simulink model "equation"  (R2025a)
settings: Solver=VariableStepAuto  StartTime=0.0  StopTime=10.0  RelTol=1e-3
settings Model: Creator=Johan  LastModifiedBy=Johan

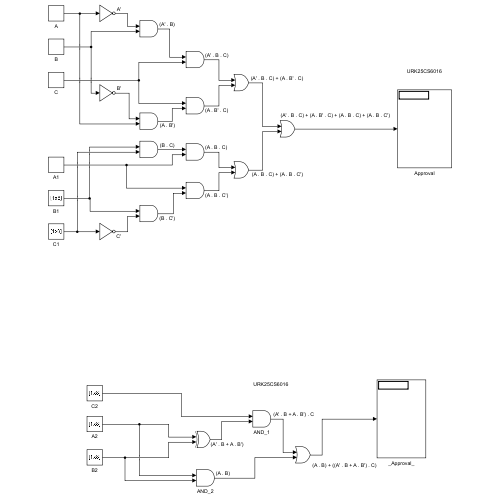
[thumbnail: Simulink's stored preview of the top-level diagram]
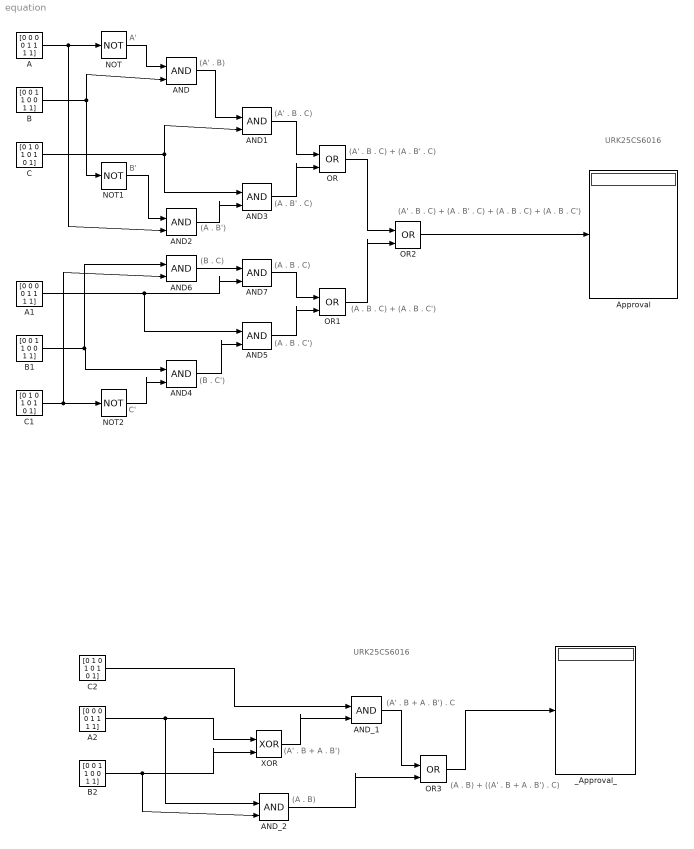
== system equation ==
  note: (A . B) + ((A' . B + A . B') . C)
  note: (A' . B + A . B') . C
  note: (A . B)
  note: (A' . B + A . B')
  note: (A' . B . C) + (A . B' . C) + (A . B . C) + (A . B . C')
  note: (A . B . C) + (A . B . C')
  note: (B . C)
  note: (B . C')
  note: (A' . B . C) + (A . B' . C)
  note: (A . B')
  note: B'
  note: (A' . B . C)
  note: (A' . B)
  note: A'
  note: URK25CS6016
  note: (A . B' . C)
  note: C'
  note: (A . B . C')
  note: (A . B . C)
  note: URK25CS6016
  A : Constant  Value=[0 0 0 0 1 1 1 1]
  A1 : Constant  Value=[0 0 0 0 1 1 1 1]
  A2 : Constant  Value=[0 0 0 0 1 1 1 1]
  AND{,1..7} (8 alike) : Logic  IconShape=distinctive  AllPortsSameDT=off  OutDataTypeStr=boolean
  AND_1 : Logic  IconShape=distinctive  AllPortsSameDT=off  OutDataTypeStr=boolean
  AND_2 : Logic  IconShape=distinctive  AllPortsSameDT=off  OutDataTypeStr=boolean
  Approval : Display
  B : Constant  Value=[0 0 1 1 0 0 1 1]
  B1 : Constant  Value=[0 0 1 1 0 0 1 1]
  B2 : Constant  Value=[0 0 1 1 0 0 1 1]
  C : Constant  Value=[0 1 0 1 0 1 0 1]
  C1 : Constant  Value=[0 1 0 1 0 1 0 1]
  C2 : Constant  Value=[0 1 0 1 0 1 0 1]
  NOT : Logic  Operator=NOT  IconShape=distinctive  AllPortsSameDT=off  OutDataTypeStr=boolean
  NOT1 : Logic  Operator=NOT  IconShape=distinctive  AllPortsSameDT=off  OutDataTypeStr=boolean
  NOT2 : Logic  Operator=NOT  IconShape=distinctive  AllPortsSameDT=off  OutDataTypeStr=boolean
  OR{,1..3} (4 alike) : Logic  Operator=OR  IconShape=distinctive  AllPortsSameDT=off  OutDataTypeStr=boolean
  XOR : Logic  Operator=XOR  IconShape=distinctive  AllPortsSameDT=off  OutDataTypeStr=boolean
  _Approval_ : Display
  wires:
  A/1 -> AND2/2, NOT/1
  NOT/1 -> AND/1
  B/1 -> NOT1/1, AND/2
  AND/1 -> AND1/1
  C/1 -> AND3/1, AND1/2
  NOT1/1 -> AND2/1
  AND2/1 -> AND3/2
  C1/1 -> NOT2/1, AND6/2
  NOT2/1 -> AND4/2
  B1/1 -> AND6/1, AND4/1
  AND4/1 -> AND5/2
  A1/1 -> AND7/2, AND5/1
  AND6/1 -> AND7/1
  AND1/1 -> OR/1
  AND3/1 -> OR/2
  AND7/1 -> OR1/1
  AND5/1 -> OR1/2
  OR/1 -> OR2/1
  OR1/1 -> OR2/2
  OR2/1 -> Approval/1
  C2/1 -> AND_1/1
  AND_1/1 -> OR3/1
  OR3/1 -> _Approval_/1
  B2/1 -> AND_2/2, XOR/2
  A2/1 -> XOR/1, AND_2/1
  XOR/1 -> AND_1/2
  AND_2/1 -> OR3/2
